simulink model "ESP_RTW"  (Simulink 8.7)
settings: Solver=ode1  SolverMode=SingleTasking  StartTime=0.0  StopTime=inf  FixedStep=0.001  RelTol=1e-3
PreLoadFcn:
  | vehicle = 'Car'; if ~length(which('cmcmd')), cmenv; end
  | ESP_RTW_bus
  | ESP_RTW_params
InitFcn:
  | vehicle = 'Car'; if ~length(which('cmcmd')), cmenv; end
  | ESP_RTW_bus
  | ESP_RTW_params
undefined symbols (not defined in the file): Area_Front, Area_Rear, ay_max_off, ay_max_on, ay_per_mu_max_off, ay_per_mu_max_on, Brake_ratio, brake_valve_ctrl_kP, cat1mode1_higher, cat1mode1_lower, cat1mode2_higher, cat1mode2_lower, cat1mode3_higher, cat1mode3_lower, cat2mode1_higher, cat2mode1_lower, cat2mode2_higher, cat2mode2_lower, cat2mode3_higher, cat2mode3_lower, delta_vel, diff_lock_fac, diff_lock_off, diff_lock_on, ESP_ctrl_kD, ESP_ctrl_kI, ESP_ctrl_kP, ESP_ctrl_restore_kI, ESP_min_throttle_fac, f_ax, f_slip, g, higherlimit_highvel, higherlimit_lowvel, highervel_fac, highervelocity_fac, InitialConditionForIntegrator, limit_acc, limit_selectlow, limit_starting, limit_vdiff, locktime_throttle, lowerlimit_highvel, lowerlimit_lowvel, lowervel_fac, lowervelocity_fac, min_throttle, MPS2KMPH, MSR_ctrl_kD, MSR_ctrl_kI, MSR_ctrl_kP, MSR_min_throttle_fac, PID_kD_sideslip, PID_kD_yawrate, PID_kI_sideslip, PID_kI_yawrate, PID_kP_sideslip, PID_kP_yawrate, RADpS2RpM, rBrake ... (+37)
libraries: CarMaker4SL x133, simulink x47, simulink_extras x6
(part 2 of 4)

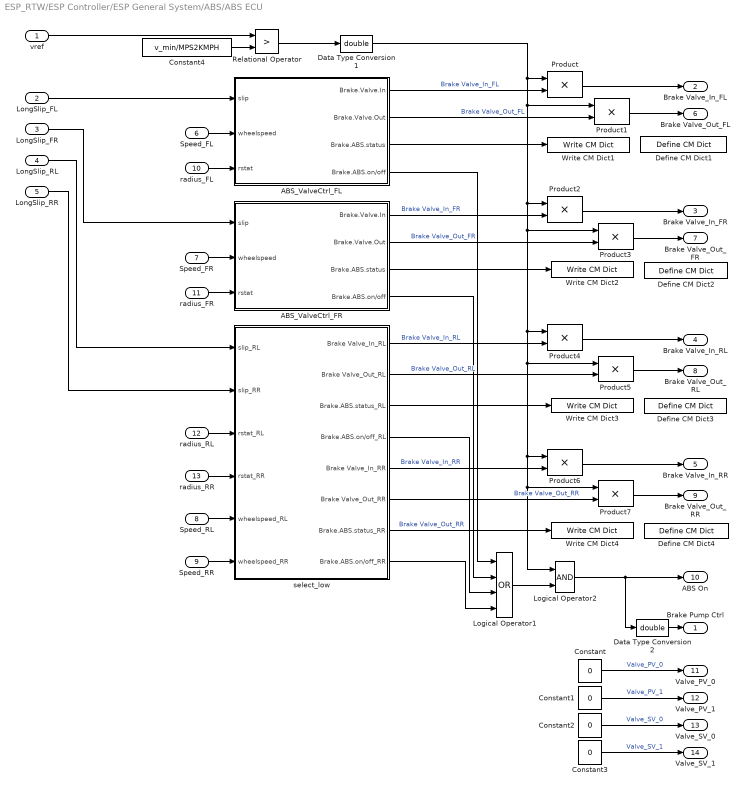
== system ESP_RTW/ESP Controller/ESP General System/ABS/ABS ECU ==
  vref : Inport
  LongSlip_FL : Inport  Port=2
  LongSlip_FR : Inport  Port=3
  LongSlip_RL : Inport  Port=4
  LongSlip_RR : Inport  Port=5
  Speed_FL : Inport  Port=6
  Speed_FR : Inport  Port=7
  Speed_RL : Inport  Port=8
  Speed_RR : Inport  Port=9
  radius_FL : Inport  Port=10
  radius_FR : Inport  Port=11
  radius_RL : Inport  Port=12
  radius_RR : Inport  Port=13
  ABS_ValveCtrl_FL : Subsystem
  ABS_ValveCtrl_FR : Subsystem
  Constant{,1..3} (4 alike) : Constant  Value=0
  Constant4 : Constant  Value=v_min/MPS2KMPH
  Data Type Conversion1 : DataTypeConversion  OutDataTypeStr=double
  Data Type Conversion2 : DataTypeConversion  OutDataTypeStr=double
  Define CM Dict1 : CarMaker4SL/Define CM Dict  xname=ESP.ABS.Status_FL  xmono=off  xtype=Char  xdvaplace=None  xnstates=4  xfirststate=0  xinitial=0
  Define CM Dict2 : CarMaker4SL/Define CM Dict  xname=ESP.ABS.Status_FR  xmono=off  xtype=Char  xdvaplace=None  xnstates=4  xfirststate=0  xinitial=0
  Define CM Dict3 : CarMaker4SL/Define CM Dict  xname=ESP.ABS.Status_RL  xmono=off  xtype=Char  xdvaplace=None  xnstates=4  xfirststate=0  xinitial=0
  Define CM Dict4 : CarMaker4SL/Define CM Dict  xname=ESP.ABS.Status_RR  xmono=off  xtype=Char  xdvaplace=None  xnstates=4  xfirststate=0  xinitial=0
  Logical Operator1 : Logic  Operator=OR  Inputs=4  AllPortsSameDT=off
  Logical Operator2 : Logic  AllPortsSameDT=off
  Product{,1..7} (8 alike) : Product  SaturateOnIntegerOverflow=on  OutDataTypeStr=Inherit: Same as first input
  Relational Operator : RelationalOperator  Operator=>
  Write CM Dict1 : CarMaker4SL/Write CM Dict  xname=ESP.ABS.Status_FL  xsync=off
  Write CM Dict2 : CarMaker4SL/Write CM Dict  xname=ESP.ABS.Status_FR  xsync=off
  Write CM Dict3 : CarMaker4SL/Write CM Dict  xname=ESP.ABS.Status_RL  xsync=off
  Write CM Dict4 : CarMaker4SL/Write CM Dict  xname=ESP.ABS.Status_RR  xsync=off
  select_low : Subsystem
  Brake Pump Ctrl : Outport
  Brake Valve_In_FL : Outport  Port=2
  Brake Valve_In_FR : Outport  Port=3
  Brake Valve_In_RL : Outport  Port=4
  Brake Valve_In_RR : Outport  Port=5
  Brake Valve_Out_FL : Outport  Port=6
  Brake Valve_Out_FR : Outport  Port=7
  Brake Valve_Out_RL : Outport  Port=8
  Brake Valve_Out_RR : Outport  Port=9
  ABS On : Outport  Port=10
  Valve_PV_0 : Outport  Port=11
  Valve_PV_1 : Outport  Port=12
  Valve_SV_0 : Outport  Port=13
  Valve_SV_1 : Outport  Port=14
  wires:
  Logical Operator2/1 -> Data Type Conversion2/1, ABS On/1
  Logical Operator1/1 -> Logical Operator2/2
  Constant3/1 -> Valve_SV_1/1  "Valve_SV_1"
  Constant2/1 -> Valve_SV_0/1  "Valve_SV_0"
  Constant1/1 -> Valve_PV_1/1  "Valve_PV_1"
  Constant/1 -> Valve_PV_0/1  "Valve_PV_0"
  vref/1 -> Relational Operator/1
  Speed_RR/1 -> select_low/6(wheelspeed_RR)
  Speed_RL/1 -> select_low/5(wheelspeed_RL)
  radius_RR/1 -> select_low/4(rstat_RR)
  radius_RL/1 -> select_low/3(rstat_RL)
  radius_FR/1 -> ABS_ValveCtrl_FR/3(rstat)
  Speed_FR/1 -> ABS_ValveCtrl_FR/2(wheelspeed)
  radius_FL/1 -> ABS_ValveCtrl_FL/3(rstat)
  Speed_FL/1 -> ABS_ValveCtrl_FL/2(wheelspeed)
  Product2/1 -> Brake Valve_In_FR/1
  Product/1 -> Brake Valve_In_FL/1
  ABS_ValveCtrl_FL/3(Brake.ABS.status) -> Write CM Dict1/1
  LongSlip_RR/1 -> select_low/2(slip_RR)
  LongSlip_RL/1 -> select_low/1(slip_RL)
  LongSlip_FR/1 -> ABS_ValveCtrl_FR/1(slip)
  LongSlip_FL/1 -> ABS_ValveCtrl_FL/1(slip)
  Product1/1 -> Brake Valve_Out_FL/1
  Product3/1 -> Brake Valve_Out_FR/1
  Product4/1 -> Brake Valve_In_RL/1
  Product5/1 -> Brake Valve_Out_RL/1
  Product6/1 -> Brake Valve_In_RR/1
  Product7/1 -> Brake Valve_Out_RR/1
  select_low/6(Brake Valve_Out_RR) -> Product7/2  "Brake Valve_Out_RR"
  select_low/5(Brake Valve_In_RR) -> Product6/2  "Brake Valve_In_RR"
  select_low/2(Brake Valve_Out_RL) -> Product5/2  "Brake Valve_Out_RL"
  select_low/1(Brake Valve_In_RL) -> Product4/2  "Brake Valve_In_RL"
  ABS_ValveCtrl_FR/2(Brake.Valve.Out) -> Product3/2  "Brake Valve_Out_FR"
  ABS_ValveCtrl_FR/1(Brake.Valve.In) -> Product2/2  "Brake Valve_In_FR"
  ABS_ValveCtrl_FL/2(Brake.Valve.Out) -> Product1/2  "Brake Valve_Out_FL"
  ABS_ValveCtrl_FL/1(Brake.Valve.In) -> Product/2  "Brake Valve_In_FL"
  Relational Operator/1 -> Data Type Conversion1/1
  Constant4/1 -> Relational Operator/2
  select_low/8(Brake.ABS.on/off_RR) -> Logical Operator1/4
  select_low/4(Brake.ABS.on/off_RL) -> Logical Operator1/3
  ABS_ValveCtrl_FR/4(Brake.ABS.on/off) -> Logical Operator1/2
  ABS_ValveCtrl_FL/4(Brake.ABS.on/off) -> Logical Operator1/1
  ABS_ValveCtrl_FR/3(Brake.ABS.status) -> Write CM Dict2/1
  select_low/3(Brake.ABS.status_RL) -> Write CM Dict3/1
  select_low/7(Brake.ABS.status_RR) -> Write CM Dict4/1  "Brake Valve_Out_RR"
  Data Type Conversion1/1 -> Product1/1, Product2/1, Product3/1, Product4/1, Product5/1, Logical Operator2/1, Product7/1, Product6/1, Product/1
  Data Type Conversion2/1 -> Brake Pump Ctrl/1

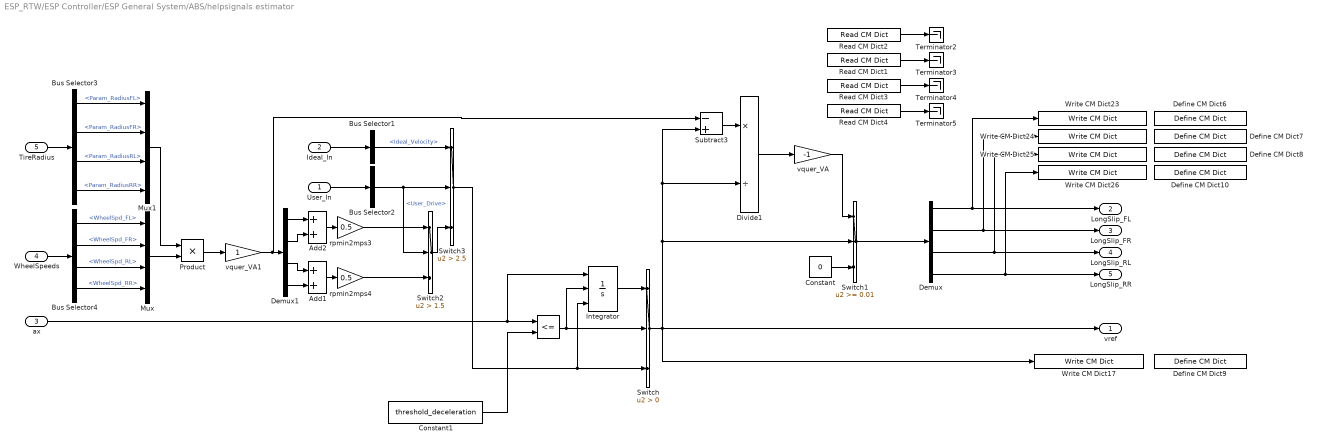
== system ESP_RTW/ESP Controller/ESP General System/ABS/helpsignals estimator ==
  User_In : Inport
  Ideal_In : Inport  Port=2
  ax : Inport  Port=3
  WheelSpeeds : Inport  Port=4
  TireRadius : Inport  Port=5
  " " : RelationalOperator  Operator=<=  OutDataTypeStr=boolean
  Add1 : Sum
  Add2 : Sum
  Bus Selector1 : BusSelector  OutputSignals=Ideal_Velocity.Ideal_Velocity
  Bus Selector2 : BusSelector  OutputSignals=User_Drive
  Bus Selector3 : BusSelector  OutputSignals=Param_RadiusFL,Param_RadiusFR,Param_RadiusRL,Param_RadiusRR
  Bus Selector4 : BusSelector  OutputSignals=WheelSpd_FL,WheelSpd_FR,WheelSpd_RL,WheelSpd_RR
  Constant : Constant  Value=0
  Constant1 : Constant  Value=threshold_deceleration
  Define CM Dict10 : CarMaker4SL/Define CM Dict  xname=ESP.ABS.LongSlip_RR  xmono=off  xtype=Double4  xdvaplace=VC  xnstates=0  xfirststate=0  xinitial=0
  Define CM Dict6 : CarMaker4SL/Define CM Dict  xname=ESP.ABS.LongSlip_FL  xmono=off  xtype=Double4  xdvaplace=VC  xnstates=0  xfirststate=0  xinitial=0
  Define CM Dict7 : CarMaker4SL/Define CM Dict  xname=ESP.ABS.LongSlip_FR  xmono=off  xtype=Double4  xdvaplace=VC  xnstates=0  xfirststate=0  xinitial=0
  Define CM Dict8 : CarMaker4SL/Define CM Dict  xname=ESP.ABS.LongSlip_RL  xmono=off  xtype=Double4  xdvaplace=VC  xnstates=0  xfirststate=0  xinitial=0
  Define CM Dict9 : CarMaker4SL/Define CM Dict  xname=ESP.ABS.v_ref  xunit=m/s  xmono=off  xtype=Double4  xdvaplace=VC  xnstates=0  xfirststate=0  xinitial=0
  Demux : Demux
  Demux1 : Demux
  Divide1 : Product  Inputs=*/
  Integrator : Integrator  ExternalReset=rising  InitialConditionSource=external
  Mux : Mux
  Mux1 : Mux
  Product : Product  RndMeth=Zero
  Read CM Dict1 : CarMaker4SL/Read CM Dict  xname=Car.LongSlipFR  xsync=off
  Read CM Dict2 : CarMaker4SL/Read CM Dict  xname=Car.LongSlipFL  xsync=off
  Read CM Dict3 : CarMaker4SL/Read CM Dict  xname=Car.LongSlipRL  xsync=off
  Read CM Dict4 : CarMaker4SL/Read CM Dict  xname=Car.LongSlipRR  xsync=off
  Subtract3 : Sum  Inputs=-+
  Switch : Switch  Criteria=u2 > Threshold
  Switch1 : Switch  Threshold=0.01
  Switch2 : Switch  Criteria=u2 > Threshold  Threshold=1.5
  Switch3 : Switch  Criteria=u2 > Threshold  Threshold=2.5
  Terminator{2..5} (4 alike) : Terminator
  Write CM Dict17 : CarMaker4SL/Write CM Dict  xname=ESP.ABS.v_ref  xsync=off
  Write CM Dict23 : CarMaker4SL/Write CM Dict  xname=ESP.ABS.LongSlip_FL  xsync=off
  Write CM Dict24 : CarMaker4SL/Write CM Dict  xname=ESP.ABS.LongSlip_FR  xsync=off
  Write CM Dict25 : CarMaker4SL/Write CM Dict  xname=ESP.ABS.LongSlip_RL  xsync=off
  Write CM Dict26 : CarMaker4SL/Write CM Dict  xname=ESP.ABS.LongSlip_RR  xsync=off
  rpmin2mps3 : Gain  Gain=0.5
  rpmin2mps4 : Gain  Gain=0.5
  vquer_VA : Gain  Gain=-1
  vquer_VA1 : Gain
  vref : Outport
  LongSlip_FL : Outport  Port=2
  LongSlip_FR : Outport  Port=3
  LongSlip_RL : Outport  Port=4
  LongSlip_RR : Outport  Port=5
  wires:
  Integrator/1 -> Switch/1
  Constant1/1 -> " "/2
  rpmin2mps4/1 -> Switch2/3
  rpmin2mps3/1 -> Switch2/1
  Bus Selector4/1 -> Mux/1  "<WheelSpd_FL>"
  Bus Selector4/2 -> Mux/2  "<WheelSpd_FR>"
  Bus Selector4/3 -> Mux/3  "<WheelSpd_RL>"
  Bus Selector4/4 -> Mux/4  "<WheelSpd_RR>"
  WheelSpeeds/1 -> Bus Selector4/1
  Bus Selector3/1 -> Mux1/1  "<Param_RadiusFL>"
  Bus Selector3/4 -> Mux1/4  "<Param_RadiusRR>"
  Bus Selector3/3 -> Mux1/3  "<Param_RadiusRL>"
  Bus Selector3/2 -> Mux1/2  "<Param_RadiusFR>"
  TireRadius/1 -> Bus Selector3/1
  Ideal_In/1 -> Bus Selector1/1
  Bus Selector1/1 -> Switch3/1  "<Ideal_Velocity>"
  Switch2/1 -> Switch3/3
  Add2/1 -> rpmin2mps3/1
  Bus Selector2/1 -> Switch3/2, Switch2/2  "<User_Drive>"
  Add1/1 -> rpmin2mps4/1
  User_In/1 -> Bus Selector2/1
  Demux1/2 -> Add2/2
  Demux1/1 -> Add2/1
  Read CM Dict4/1 -> Terminator5/1
  Read CM Dict3/1 -> Terminator4/1
  Read CM Dict1/1 -> Terminator3/1
  Read CM Dict2/1 -> Terminator2/1
  " "/1 -> Switch/2, Integrator/2
  vquer_VA1/1 -> Demux1/1, Subtract3/1
  Demux/4 -> Write CM Dict26/1, LongSlip_RR/1
  Demux/3 -> Write CM Dict25/1, LongSlip_RL/1
  Demux/2 -> Write CM Dict24/1, LongSlip_FR/1
  Demux/1 -> Write CM Dict23/1, LongSlip_FL/1
  Constant/1 -> Switch1/3
  Switch1/1 -> Demux/1
  Switch/1 -> Write CM Dict17/1, vref/1, Switch1/2, Divide1/2, Subtract3/2
  Demux1/4 -> Add1/2
  Demux1/3 -> Add1/1
  Switch3/1 -> Switch/3, Integrator/3
  ax/1 -> " "/1, Integrator/1
  vquer_VA/1 -> Switch1/1
  Divide1/1 -> vquer_VA/1
  Subtract3/1 -> Divide1/1
  Mux/1 -> Product/2
  Mux1/1 -> Product/1
  Product/1 -> vquer_VA1/1

== system ESP_RTW/ESP Controller/ESP General System/ASR/BMR ECU ==
  Throttle : Inport
  WheelVelocity [kmph] : Inport  Port=2
  User_In : Inport  Port=3
  Ideal_In : Inport  Port=4
  BMR Controller : Subsystem
  BMR logic : Subsystem
  Bus Creator : BusCreator  Inputs=8
  Bus Creator1 : BusCreator  Inputs=2
  Bus Creator2 : BusCreator  Inputs=2
  Bus Creator3 : BusCreator  Inputs=2
  Differential Lock : Subsystem
  Signal Mapping : Subsystem
  BMR On : Outport
  Brake Valves : Outport  Port=2
  Pilot Valves : Outport  Port=3
  Suctions Valves : Outport  Port=4
  Pump Ctrl : Outport  Port=5
  Diff_Torque : Outport  Port=6
  wires:
  User_In/1 -> Signal Mapping/1(User_In), Differential Lock/1(User_In), BMR Controller/1(User_In)
  BMR logic/2(BMR On) -> BMR On/1, BMR Controller/3(BMR On)
  BMR logic/1(mode) -> BMR Controller/2(mode)
  Throttle/1 -> BMR logic/5(Throttle position)
  Signal Mapping/4(v_UndrivenR) -> BMR logic/4(v_undrivenR)
  Signal Mapping/3(v_UndrivenL) -> BMR logic/3(v_undrivenL)
  Signal Mapping/2(v_DrivenR) -> BMR logic/2(v_drivenR), Differential Lock/3(v_DrivenR)
  Signal Mapping/1(v_DrivenL) -> BMR logic/1(v_drivenL), Differential Lock/2(v_DrivenL)
  Ideal_In/1 -> Signal Mapping/3(Ideal_In)
  Bus Creator3/1 -> Diff_Torque/1
  Differential Lock/2(RearDiff_Torque) -> Bus Creator3/2  "RearDiff_Torque"
  Differential Lock/1(FrontDiff_Torque) -> Bus Creator3/1  "FrontDiff_Torque"
  WheelVelocity [kmph]/1 -> Signal Mapping/2(WheelVelocity)
  Bus Creator1/1 -> Suctions Valves/1
  Bus Creator2/1 -> Pilot Valves/1
  BMR Controller/13(Pump Ctrl) -> Pump Ctrl/1  "PumpCtrl"
  BMR Controller/12(Valve_SV_1) -> Bus Creator1/2  "Valve_SV_1"
  BMR Controller/11(Valve_SV_0) -> Bus Creator1/1  "Valve_SV_0"
  BMR Controller/10(Valve_PV_1) -> Bus Creator2/2  "Valve_PV_1"
  BMR Controller/9(Valve_PV_0) -> Bus Creator2/1  "Valve_PV_0"
  BMR Controller/8(Brake Valve_Out_RR) -> Bus Creator/8  "Valve_Out_RR"
  BMR Controller/7(Brake Valve_Out_RL) -> Bus Creator/7  "Valve_Out_RL"
  BMR Controller/6(Brake Valve_Out_FR) -> Bus Creator/6  "Valve_Out_FR"
  BMR Controller/5(Brake Valve_Out_FL) -> Bus Creator/5  "Valve_Out_FL"
  BMR Controller/4(Brake Valve_In_RR) -> Bus Creator/4  "Valve_In_RR"
  BMR Controller/3(Brake Valve_In_RL) -> Bus Creator/3  "Valve_In_RL"
  BMR Controller/2(Brake Valve_In_FR) -> Bus Creator/2  "Valve_In_FR"
  BMR Controller/1(Brake Valve_In_FL) -> Bus Creator/1  "Valve_In_FL"
  Bus Creator/1 -> Brake Valves/1

== system ESP_RTW/ESP Controller/ESP General System/ASR/MSR ECU ==
  Throttle Position : Inport
  WheelVelocity [kmph] : Inport  Port=2
  User_In : Inport  Port=3
  Ideal_In : Inport  Port=4
  MSR logic : Subsystem
  MSR/Gas Controller : Subsystem
  Signal Mapping : Subsystem
  Gas_out : Outport
  MSR On : Outport  Port=2
  wires:
  MSR logic/3(hold torque) -> MSR/Gas Controller/4(hold Gas)
  MSR logic/2(reduce torque) -> MSR/Gas Controller/3(close Gas)
  MSR logic/1(Pseudo_slip) -> MSR/Gas Controller/2(Pseudo_Slip)
  Signal Mapping/4(v_UndrivenR) -> MSR logic/4(v_undrivenR)
  Signal Mapping/3(v_UndrivenL) -> MSR logic/3(v_undrivenL)
  Signal Mapping/2(v_DrivenR) -> MSR logic/2(v_drivenR)
  Signal Mapping/1(v_DrivenL) -> MSR logic/1(v_drivenL)
  Ideal_In/1 -> Signal Mapping/3(Ideal_In)
  User_In/1 -> Signal Mapping/2(User_In)
  WheelVelocity [kmph]/1 -> Signal Mapping/1(WheelVelocity)
  MSR/Gas Controller/2(Gas_Out) -> Gas_out/1
  MSR/Gas Controller/1(MSR_On) -> MSR On/1
  Throttle Position/1 -> MSR/Gas Controller/1(Throttle_position)

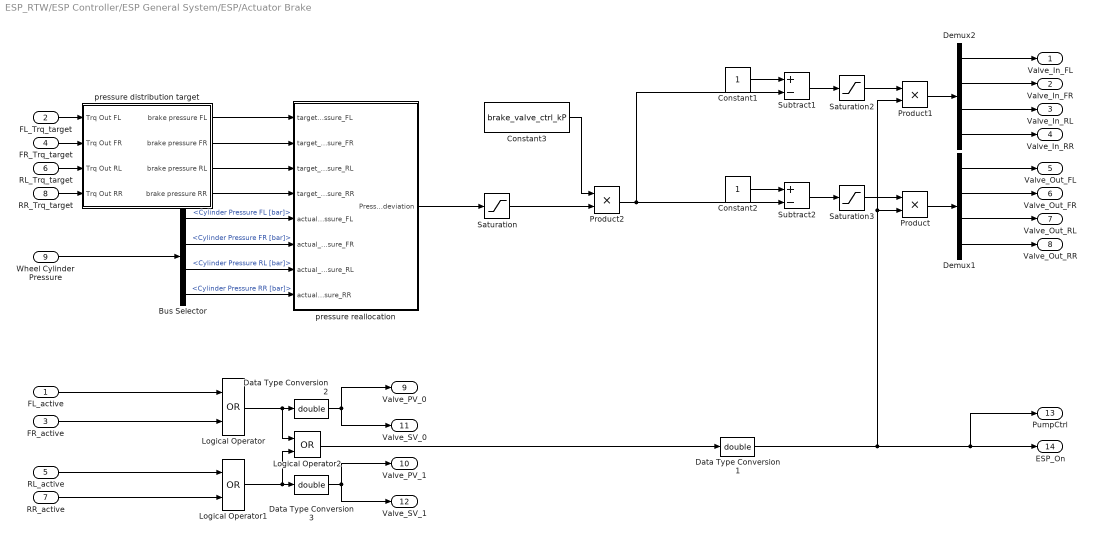
== system ESP_RTW/ESP Controller/ESP General System/ESP/Actuator Brake ==
  FL_active : Inport
  FL_Trq_target : Inport  Port=2
  FR_active : Inport  Port=3
  FR_Trq_target : Inport  Port=4
  RL_active : Inport  Port=5
  RL_Trq_target : Inport  Port=6
  RR_active : Inport  Port=7
  RR_Trq_target : Inport  Port=8
  Wheel Cylinder Pressure : Inport  Port=9
  Bus Selector : BusSelector  OutputSignals=Cylinder Pressure FL [bar],Cylinder Pressure FR [bar],Cylinder Pressure RL [bar],Cylinder Pressure RR [bar]
  Constant1 : Constant
  Constant2 : Constant
  Constant3 : Constant  Value=brake_valve_ctrl_kP
  Data Type Conversion1 : DataTypeConversion  OutDataTypeStr=double
  Data Type Conversion2 : DataTypeConversion  OutDataTypeStr=double
  Data Type Conversion3 : DataTypeConversion  OutDataTypeStr=double
  Demux1 : Demux
  Demux2 : Demux
  Logical Operator : Logic  Operator=OR  AllPortsSameDT=off
  Logical Operator1 : Logic  Operator=OR  AllPortsSameDT=off
  Logical Operator2 : Logic  Operator=OR  AllPortsSameDT=off
  Product : Product  RndMeth=Zero
  Product1 : Product  RndMeth=Zero
  Product2 : Product  RndMeth=Zero
  Saturation : Saturate  UpperLimit=500  LowerLimit=0
  Saturation2 : Saturate  UpperLimit=1  LowerLimit=0
  Saturation3 : Saturate  UpperLimit=1  LowerLimit=0
  Subtract1 : Sum  Inputs=+-
  Subtract2 : Sum  Inputs=+-
  pressure distribution target : Subsystem
  pressure reallocation : Subsystem
  Valve_In_FL : Outport
  Valve_In_FR : Outport  Port=2
  Valve_In_RL : Outport  Port=3
  Valve_In_RR : Outport  Port=4
  Valve_Out_FL : Outport  Port=5
  Valve_Out_FR : Outport  Port=6
  Valve_Out_RL : Outport  Port=7
  Valve_Out_RR : Outport  Port=8
  Valve_PV_0 : Outport  Port=9
  Valve_PV_1 : Outport  Port=10
  Valve_SV_0 : Outport  Port=11
  Valve_SV_1 : Outport  Port=12
  PumpCtrl : Outport  Port=13
  ESP_On : Outport  Port=14
  wires:
  pressure reallocation/1(Pressure deviation) -> Saturation/1
  Bus Selector/4 -> pressure reallocation/8(actual_pressure_RR)  "<Cylinder Pressure RR [bar]>"
  Bus Selector/3 -> pressure reallocation/7(actual_pressure_RL)  "<Cylinder Pressure RL [bar]>"
  Bus Selector/2 -> pressure reallocation/6(actual_pressure_FR)  "<Cylinder Pressure FR [bar]>"
  Bus Selector/1 -> pressure reallocation/5(actual_pressure_FL)  "<Cylinder Pressure FL [bar]>"
  pressure distribution target/4(brake pressure RR) -> pressure reallocation/4(target_pressure_RR)
  pressure distribution target/3(brake pressure RL) -> pressure reallocation/3(target_pressure_RL)
  pressure distribution target/2(brake pressure FR) -> pressure reallocation/2(target_pressure_FR)
  pressure distribution target/1(brake pressure FL) -> pressure reallocation/1(target_pressure_FL)
  Constant3/1 -> Product2/1
  Wheel Cylinder Pressure/1 -> Bus Selector/1
  Product1/1 -> Demux2/1
  Saturation2/1 -> Product1/1
  Product/1 -> Demux1/1
  Saturation3/1 -> Product/1
  Demux2/4 -> Valve_In_RR/1
  Demux2/3 -> Valve_In_RL/1
  Demux2/2 -> Valve_In_FR/1
  Demux2/1 -> Valve_In_FL/1
  Demux1/4 -> Valve_Out_RR/1
  Demux1/3 -> Valve_Out_RL/1
  RR_Trq_target/1 -> pressure distribution target/4(Trq Out RR)
  RL_Trq_target/1 -> pressure distribution target/3(Trq Out RL)
  Demux1/2 -> Valve_Out_FR/1
  Demux1/1 -> Valve_Out_FL/1
  Subtract2/1 -> Saturation3/1
  Subtract1/1 -> Saturation2/1
  Logical Operator2/1 -> Data Type Conversion1/1
  Logical Operator1/1 -> Logical Operator2/2, Data Type Conversion3/1
  RR_active/1 -> Logical Operator1/2
  RL_active/1 -> Logical Operator1/1
  Logical Operator/1 -> Logical Operator2/1, Data Type Conversion2/1
  FR_active/1 -> Logical Operator/2
  FL_active/1 -> Logical Operator/1
  FR_Trq_target/1 -> pressure distribution target/2(Trq Out FR)
  Constant2/1 -> Subtract2/1
  Constant1/1 -> Subtract1/1
  Saturation/1 -> Product2/2
  Product2/1 -> Subtract1/2, Subtract2/2
  FL_Trq_target/1 -> pressure distribution target/1(Trq Out FL)
  Data Type Conversion1/1 -> Product/2, Product1/2, PumpCtrl/1, ESP_On/1
  Data Type Conversion2/1 -> Valve_SV_0/1, Valve_PV_0/1
  Data Type Conversion3/1 -> Valve_SV_1/1, Valve_PV_1/1

== system ESP_RTW/ESP Controller/ESP General System/ESP/ECU ==
  ax : Inport
  Throttle Position : Inport  Port=2
  Yaw Rate : Inport  Port=3
  Steer Angle : Inport  Port=4
  Sideslip : Inport  Port=5
  mu : Inport  Port=6
  ay : Inport  Port=7
  Ideal_In : Inport  Port=8
  Vehicle Params : Inport  Port=9
  User_In : Inport  Port=10
  ECU logic : Subsystem
  Instability detectors : Subsystem
  Motor management strategy : Subsystem
  brake distribution strategy : Subsystem
  Gas_out : Outport
  FL_active : Outport  Port=2
  FL_Trq_target : Outport  Port=3
  FR_active : Outport  Port=4
  FR_Trq_target : Outport  Port=5
  RL_active : Outport  Port=6
  RL_Trq_target : Outport  Port=7
  RR_active : Outport  Port=8
  RR_Trq_target : Outport  Port=9
  wires:
  User_In/1 -> brake distribution strategy/4(User_In)
  Vehicle Params/1 -> brake distribution strategy/3(Vehicle Params), Instability detectors/7(Vehicle Params)
  Ideal_In/1 -> Instability detectors/6(Ideal_In), ECU logic/4(Ideal_In)
  mu/1 -> Instability detectors/5(mu_max), ECU logic/3(mu_max)
  Sideslip/1 -> Instability detectors/4(Sideslip)
  Instability detectors/3(motormanagement activation) -> Motor management strategy/1(activation DK)
  ay/1 -> Instability detectors/3(ay)
  Motor management strategy/1(Gas_out) -> Gas_out/1
  ax/1 -> Motor management strategy/3(ax)
  Throttle Position/1 -> Motor management strategy/2(Throttle_position)
  Instability detectors/2(YawRate corrected deviation) -> ECU logic/2(YawRate corrected deviation)
  Instability detectors/1(SideSlipAngle deviation) -> ECU logic/1(SideSlipAngle deviation)
  brake distribution strategy/8(Trq_RR_target) -> RR_Trq_target/1
  brake distribution strategy/7(RR_active) -> RR_active/1
  brake distribution strategy/6(Trq_RL_target) -> RL_Trq_target/1
  brake distribution strategy/5(RL_active) -> RL_active/1
  brake distribution strategy/4(Trq_FR_target) -> FR_Trq_target/1
  brake distribution strategy/3(FR_active) -> FR_active/1
  brake distribution strategy/2(Trq_FL_target) -> FL_Trq_target/1
  brake distribution strategy/1(FL_active) -> FL_active/1
  Yaw Rate/1 -> Instability detectors/2(Yaw Rate)
  Steer Angle/1 -> brake distribution strategy/1(Steer Angle), Instability detectors/1(Steer Angle)
  ECU logic/1(Stabilizing Torque) -> brake distribution strategy/2(Stabilizing Torque)

== system ESP_RTW/ESP Controller/ESP General System/ESP/helpsignals estimator ==
  Steer Angle : Inport
  Ideal_In : Inport  Port=2
  Vehicle Params : Inport  Port=3
  User_In : Inport  Port=4
  Bus Selector1 : BusSelector  OutputSignals=Ideal_SideSlipAngle
  Bus Selector2 : BusSelector  OutputSignals=User_estimators_on.User_SideSlip_estimator_on,User_estimators_on.User_mue_estimator_on
  Bus Selector3 : BusSelector  OutputSignals=Ideal_mu.Ideal_muFL,Ideal_mu.Ideal_muFR,Ideal_mu.Ideal_muRL,Ideal_mu.Ideal_muRR
  MinMax : MinMax  Inputs=4
  SideSlip estimator : Subsystem
  Switch : Switch  Criteria=u2 > Threshold
  Switch1 : Switch  Criteria=u2 > Threshold
  mue estimator : Subsystem
  SideslipAngle : Outport
  mu : Outport  Port=2
  wires:
  Vehicle Params/1 -> mue estimator/2(Vehicle Params)
  Bus Selector3/1 -> MinMax/1  "<Ideal_muFL>"
  Bus Selector3/4 -> MinMax/4  "<Ideal_muRR>"
  Bus Selector3/2 -> MinMax/2  "<Ideal_muFR>"
  Bus Selector3/3 -> MinMax/3  "<Ideal_muRL>"
  Ideal_In/1 -> Bus Selector1/1, SideSlip estimator/2(CarMaker_In), mue estimator/1(CarMaker_In), Bus Selector3/1
  MinMax/1 -> Switch1/3
  Switch1/1 -> mu/1
  Bus Selector2/2 -> Switch1/2  "<User_mue_estimator_on>"
  Switch/1 -> SideslipAngle/1
  SideSlip estimator/1(SideSlipAngle_estimated) -> Switch/1
  Bus Selector1/1 -> Switch/3  "<Ideal_SideSlipAngle>"
  Bus Selector2/1 -> Switch/2  "<User_SideSlip_estimator_on>"
  User_In/1 -> Bus Selector2/1
  mue estimator/1(mue_estimated) -> Switch1/1
  Steer Angle/1 -> SideSlip estimator/1(lenkwinkel)

== system ESP_RTW/ESP Controller/ESP General System/Master Controller/ABS Off ==
  ABS On : Inport
  ABS Bus : Inport  Port=2
  Bus Creator : BusCreator  Inputs=8
  Bus Creator4 : BusCreator  Inputs='Pilot Valves','Suction Valves','Brake Valves','Pump Ctrl'
  Bus Selector1 : BusSelector  OutputSignals=Valve_In_FL,Valve_In_FR,Valve_In_RL,Valve_In_RR,Valve_Out_FL,Valve_Out_FR,Valve_Out_RL,Valve_Out_RR
  Bus Selector3 : BusSelector  OutputSignals=Pilot Valves,Suction Valves,Brake Valves,Pump Ctrl
  Product{,1..7} (8 alike) : Product  RndMeth=Zero
  ABS Bus Out : Outport
  wires:
  Product7/1 -> Bus Creator/8  "Valve_Out_RR"
  Bus Selector1/8 -> Product7/2  "<Valve_Out_RR>"
  Product6/1 -> Bus Creator/7  "Valve_Out_RL"
  Bus Selector1/7 -> Product6/2  "<Valve_Out_RL>"
  Product5/1 -> Bus Creator/6  "Valve_Out_FR"
  Bus Selector1/6 -> Product5/2  "<Valve_Out_FR>"
  Product4/1 -> Bus Creator/5  "Valve_Out_FL"
  Bus Selector1/5 -> Product4/2  "<Valve_Out_FL>"
  Product3/1 -> Bus Creator/4  "Valve_In_RR"
  Bus Selector1/4 -> Product3/2  "<Valve_In_RR>"
  Product2/1 -> Bus Creator/3  "Valve_In_RL"
  Bus Selector1/3 -> Product2/2  "<Valve_In_RL>"
  Product1/1 -> Bus Creator/2  "Valve_In_FR"
  Bus Selector1/2 -> Product1/2  "<Valve_In_FR>"
  Product/1 -> Bus Creator/1  "Valve_In_FL"
  Bus Selector1/1 -> Product/2  "<Valve_In_FL>"
  ABS On/1 -> Product/1, Product1/1, Product2/1, Product3/1, Product4/1, Product5/1, Product6/1, Product7/1
  Bus Creator/1 -> Bus Creator4/3  "Brake Valves"
  Bus Selector3/4 -> Bus Creator4/4  "<Pump Ctrl>"
  Bus Selector3/3 -> Bus Selector1/1  "<Brake Valves>"
  Bus Selector3/2 -> Bus Creator4/2  "<Suction Valves>"
  Bus Selector3/1 -> Bus Creator4/1  "<Pilot Valves>"
  ABS Bus/1 -> Bus Selector3/1
  Bus Creator4/1 -> ABS Bus Out/1  "ABS Bus"

== system ESP_RTW/ESP Controller/ESP General System/Master Controller/Actuator VC ==
  VC_IN : Inport
  HSA_BrakePark : Inport  Port=2
  Gas_Out_ASR : Inport  Port=3
  Gas_Out_ESP : Inport  Port=4
  HSA_Flag : Inport  Port=5
  ASR_Flag : Inport  Port=6
  ESP_Flag : Inport  Port=7
  Bus Selector3 : BusSelector  OutputSignals=Gas,Park
  Bus Creator : BusCreator  Inputs=2
  Constant : Constant
  MinMax : MinMax  Inputs=3
  MinMax1 : MinMax  Function=max  Inputs=2
  Product : Product  RndMeth=Zero
  Subtract1 : Sum  Inputs=+-+
  Subtract2 : Sum  Inputs=+-+
  VC_OUT : Outport
  wires:
  ESP_Flag/1 -> Subtract2/2
  MinMax/1 -> Bus Creator/1  "VC_Gas"
  Bus Creator/1 -> VC_OUT/1
  MinMax1/1 -> Bus Creator/2  "VC_BrakePark"
  Product/1 -> MinMax1/2
  HSA_BrakePark/1 -> Product/2
  HSA_Flag/1 -> Product/1
  Bus Selector3/2 -> MinMax1/1  "<Park>"
  Bus Selector3/1 -> MinMax/3  "<Gas>"
  VC_IN/1 -> Bus Selector3/1
  Subtract1/1 -> MinMax/2
  Gas_Out_ASR/1 -> Subtract1/3
  ASR_Flag/1 -> Subtract1/2
  Subtract2/1 -> MinMax/1
  Gas_Out_ESP/1 -> Subtract2/3
  Constant/1 -> Subtract2/1, Subtract1/1

== system ESP_RTW/ESP Controller/ESP General System/Master Controller/User Switch ==
  ESP On : Inport
  ASR On : Inport  Port=2
  ABS On : Inport  Port=3
  HSA On : Inport  Port=4
  User In : Inport  Port=5
  Bus Creator6 : BusCreator  Inputs=3
  Bus Selector : BusSelector  OutputSignals=ASR On,MSR On,BMR On
  Bus Selector4 : BusSelector  OutputSignals=User_Switch.User_Switch_Main_off,User_Switch.User_Switch_ESP_off,User_Switch.User_Switch_ASR_off,User_Switch.User_Switch_ABS_off,User_Switch.User_Switch_HSA_off
  Constant : Constant
  Product{,1..9} (10 alike) : Product  RndMeth=Zero
  Subtract{,1..4} (5 alike) : Sum  Inputs=+-
  "ESP On " : Outport
  "ASR On " : Outport  Port=2
  "ABS On " : Outport  Port=3
  "HSA On " : Outport  Port=4
  ASRASR On : Outport  Port=5
  wires:
  Product9/1 -> "HSA On "/1  "HSA On"
  HSA On/1 -> Product9/2
  Product8/1 -> Product9/1
  Subtract4/1 -> Product8/2
  Bus Selector4/5 -> Subtract4/2  "<User_Switch_HSA_off>"
  User In/1 -> Bus Selector4/1
  Product7/1 -> "ABS On "/1  "ABS On"
  ABS On/1 -> Product7/2
  Product2/1 -> Product7/1
  Product6/1 -> Bus Creator6/3  "BMR On"
  Bus Selector/3 -> Product6/2  "<BMR On>"
  Bus Creator6/1 -> "ASR On "/1  "ASR On"
  Product5/1 -> Bus Creator6/2  "MSR On"
  Bus Selector/2 -> Product5/2  "<MSR On>"
  Product4/1 -> ASRASR On/1, Bus Creator6/1  "ASR On"
  Bus Selector/1 -> Product4/2  "<ASR On>"
  Product1/1 -> Product4/1, Product5/1, Product6/1
  Product3/1 -> "ESP On "/1  "ESP On"
  ESP On/1 -> Product3/2
  Product/1 -> Product3/1
  Subtract3/1 -> Product2/2
  Subtract2/1 -> Product1/2
  Subtract1/1 -> Product/2
  Subtract/1 -> Product2/1, Product8/1, Product1/1, Product/1
  Bus Selector4/4 -> Subtract3/2  "<User_Switch_ABS_off>"
  Bus Selector4/3 -> Subtract2/2  "<User_Switch_ASR_off>"
  Bus Selector4/2 -> Subtract1/2  "<User_Switch_ESP_off>"
  Bus Selector4/1 -> Subtract/2  "<User_Switch_Main_off>"
  Constant/1 -> Subtract/1, Subtract1/1, Subtract2/1, Subtract3/1, Subtract4/1
  ASR On/1 -> Bus Selector/1

== system ESP_RTW/ESP Controller/ESP General System/ABS/ABS ECU/ABS_ValveCtrl_FL ==
  note: EITHER ABS is switched on and  S_K is put through
      |  when S_K is becomming bigger the s_{ku}
      | OR output is 0 when S_K is smaller than {sku}_{off}
  note: Valve Control:
      | Valves are open for a predefined time window.
      | The driving time depends on a trigger criterion (LUT).
      | The treshold change for the valve driving time is
      | continously modified by a repeating sequence.
  note: Control strategy: Trigger criterion S_K
      | S_K combines wheel decceleration control with slip control
      | using weighting factors  K_z and K_\lambda
      | S_K=K_z*z_R + K_\lambda * \lambda_{rel}
      | (see p.127 in M. Burckhardt
      | Fahrwerktechnik:Radschlupfregelsysteme)
  slip : Inport
  wheelspeed : Inport  Port=2
  rstat : Inport  Port=3
  Constant : Constant
  Constant1 : Constant  Value=f_slip
  Constant3 : Constant  Value=f_ax
  Derivative : Derivative
  Duty : Subsystem
  Look-Up Table1 : Lookup  InputValues=Valve_LUTin_VA  Table=ValveIn_LUTout_VA  LookUpMeth=Interpolation-Use End Values  SaturateOnIntegerOverflow=on
  Look-Up Table2 : Lookup  InputValues=Valve_LUTin_VA  Table=ValveOut_LUTout_VA  LookUpMeth=Interpolation-Use End Values  SaturateOnIntegerOverflow=on
  Product : Product  SaturateOnIntegerOverflow=on  OutDataTypeStr=Inherit: Same as first input
  Product1 : Product  Inputs=3  SaturateOnIntegerOverflow=on  InputSameDT=on  OutDataTypeStr=Inherit: Same as first input
  Product2 : Product  SaturateOnIntegerOverflow=on  OutDataTypeStr=Inherit: Same as first input
  Rate Transition{1..4} (4 alike) : RateTransition
  Relational Operator : RelationalOperator  Operator=<  SampleTime=0.001
  Relational Operator1 : RelationalOperator  Operator=<  SampleTime=0.001
  Relay : Relay  OnSwitchValue=sku_VA  OffSwitchValue=sku_off_VA
  Sum : Sum  Inputs=|--  SaturateOnIntegerOverflow=on  InputSameDT=on  OutDataTypeStr=Inherit: Same as first input
  Sum1 : Sum  Inputs=--+  SaturateOnIntegerOverflow=on
  Zero-Order Hold : ZeroOrderHold  SampleTime=t_Sensor
  Brake.Valve.In : Outport
  Brake.Valve.Out : Outport  Port=2
  Brake.ABS.status : Outport  Port=3
  Brake.ABS.on/off : Outport  Port=4
  wires:
  Rate Transition2/1 -> Relational Operator1/1, Relational Operator/1
  Rate Transition4/1 -> Brake.ABS.on/off/1
  Rate Transition3/1 -> Relational Operator1/2
  Rate Transition1/1 -> Relational Operator/2
  Duty/1(SZ) -> Rate Transition2/1
  Constant1/1 -> Product2/1
  Derivative/1 -> Product1/1
  Product2/1 -> Sum/1
  Product1/1 -> Sum/2
  slip/1 -> Product2/2
  wheelspeed/1 -> Derivative/1
  rstat/1 -> Product1/2
  Constant3/1 -> Product1/3
  Relational Operator/1 -> Brake.Valve.In/1, Sum1/1
  Relational Operator1/1 -> Sum1/2, Brake.Valve.Out/1
  Constant/1 -> Sum1/3
  Sum1/1 -> Brake.ABS.status/1
  Sum/1 -> Zero-Order Hold/1  "S_K"
  Product/1 -> Look-Up Table2/1, Look-Up Table1/1
  Look-Up Table1/1 -> Rate Transition1/1
  Look-Up Table2/1 -> Rate Transition3/1
  Relay/1 -> Product/2, Rate Transition4/1
  Zero-Order Hold/1 -> Relay/1, Product/1

== system ESP_RTW/ESP Controller/ESP General System/ABS/ABS ECU/ABS_ValveCtrl_FR ==
  note: EITHER ABS is switched on and  S_K is put through
      |  when S_K is becomming bigger the s_{ku}
      | OR output is 0 when S_K is smaller than {sku}_{off}
  note: Valve Control:
      | Valves are open for a predefined time window.
      | The driving time depends on a trigger criterion (LUT).
      | The treshold change for the valve driving time is
      | continously modified by a repeating sequence.
  note: Control strategy: Trigger criterion S_K
      | S_K combines wheel decceleration control with slip control
      | using weighting factors  K_z and K_\lambda
      | S_K=K_z*z_R + K_\lambda * \lambda_{rel}
      | (see p.127 in M. Burckhardt
      | Fahrwerktechnik:Radschlupfregelsysteme)
  slip : Inport
  wheelspeed : Inport  Port=2
  rstat : Inport  Port=3
  Constant : Constant
  Constant1 : Constant  Value=f_slip
  Constant3 : Constant  Value=f_ax
  Derivative : Derivative
  Duty : Subsystem
  Look-Up Table1 : Lookup  InputValues=Valve_LUTin_VA  Table=ValveIn_LUTout_VA  LookUpMeth=Interpolation-Use End Values  SaturateOnIntegerOverflow=on
  Look-Up Table2 : Lookup  InputValues=Valve_LUTin_VA  Table=ValveOut_LUTout_VA  LookUpMeth=Interpolation-Use End Values  SaturateOnIntegerOverflow=on
  Product : Product  SaturateOnIntegerOverflow=on  OutDataTypeStr=Inherit: Same as first input
  Product1 : Product  Inputs=3  SaturateOnIntegerOverflow=on  InputSameDT=on  OutDataTypeStr=Inherit: Same as first input
  Product2 : Product  SaturateOnIntegerOverflow=on  OutDataTypeStr=Inherit: Same as first input
  Rate Transition{1..4} (4 alike) : RateTransition
  Relational Operator : RelationalOperator  Operator=<  SampleTime=0.001
  Relational Operator1 : RelationalOperator  Operator=<  SampleTime=0.001
  Relay : Relay  OnSwitchValue=sku_VA  OffSwitchValue=sku_off_VA
  Sum : Sum  Inputs=|--  SaturateOnIntegerOverflow=on  InputSameDT=on  OutDataTypeStr=Inherit: Same as first input
  Sum1 : Sum  Inputs=--+  SaturateOnIntegerOverflow=on
  Zero-Order Hold : ZeroOrderHold  SampleTime=t_Sensor
  Brake.Valve.In : Outport
  Brake.Valve.Out : Outport  Port=2
  Brake.ABS.status : Outport  Port=3
  Brake.ABS.on/off : Outport  Port=4
  wires:
  Rate Transition4/1 -> Brake.ABS.on/off/1
  Rate Transition3/1 -> Relational Operator1/2
  Rate Transition1/1 -> Relational Operator/2
  Rate Transition2/1 -> Relational Operator1/1, Relational Operator/1
  Constant1/1 -> Product2/1
  Derivative/1 -> Product1/1
  Product2/1 -> Sum/1
  Product1/1 -> Sum/2
  slip/1 -> Product2/2
  wheelspeed/1 -> Derivative/1
  rstat/1 -> Product1/2
  Constant3/1 -> Product1/3
  Relational Operator/1 -> Brake.Valve.In/1, Sum1/1
  Relational Operator1/1 -> Brake.Valve.Out/1, Sum1/2
  Constant/1 -> Sum1/3
  Sum1/1 -> Brake.ABS.status/1
  Sum/1 -> Zero-Order Hold/1
  Product/1 -> Look-Up Table1/1, Look-Up Table2/1
  Duty/1(SZ) -> Rate Transition2/1
  Look-Up Table1/1 -> Rate Transition1/1
  Look-Up Table2/1 -> Rate Transition3/1
  Relay/1 -> Product/2, Rate Transition4/1
  Zero-Order Hold/1 -> Relay/1, Product/1

== system ESP_RTW/ESP Controller/ESP General System/ABS/ABS ECU/select_low ==
  note: Control strategy: Trigger criterion S_K
      | S_K combines wheel decceleration control with slip control
      | using weighting factors  K_z and K_\lambda
      | S_K=K_z*z_R + K_\lambda * \lambda_{rel}
      | (see p.127 in M. Burckhardt
      | Fahrwerktechnik:Radschlupfregelsysteme)
  slip_RL : Inport
  slip_RR : Inport  Port=2
  rstat_RL : Inport  Port=3
  rstat_RR : Inport  Port=4
  wheelspeed_RL : Inport  Port=5
  wheelspeed_RR : Inport  Port=6
  ABS_ValveCtrl_rear : Subsystem
  Constant1 : Constant  Value=f_ax
  Constant2 : Constant  Value=f_slip
  Constant3 : Constant  Value=f_ax
  Constant4 : Constant  Value=f_slip
  Derivative : Derivative
  Derivative1 : Derivative
  MinMax : MinMax  Function=max  Inputs=2  SaturateOnIntegerOverflow=on  InputSameDT=on
  Product1 : Product  Inputs=3  SaturateOnIntegerOverflow=on  InputSameDT=on  OutDataTypeStr=Inherit: Same as first input
  Product2 : Product  Inputs=3  SaturateOnIntegerOverflow=on  InputSameDT=on  OutDataTypeStr=Inherit: Same as first input
  Product3 : Product  SaturateOnIntegerOverflow=on  OutDataTypeStr=Inherit: Same as first input
  Product4 : Product  SaturateOnIntegerOverflow=on  OutDataTypeStr=Inherit: Same as first input
  Sum : Sum  Inputs=|--  SaturateOnIntegerOverflow=on  InputSameDT=on  OutDataTypeStr=Inherit: Same as first input
  Sum1 : Sum  Inputs=|--  SaturateOnIntegerOverflow=on  InputSameDT=on  OutDataTypeStr=Inherit: Same as first input
  Brake Valve_In_RL : Outport
  Brake Valve_Out_RL : Outport  Port=2
  Brake.ABS.status_RL : Outport  Port=3
  Brake.ABS.on/off_RL : Outport  Port=4
  Brake Valve_In_RR : Outport  Port=5
  Brake Valve_Out_RR : Outport  Port=6
  Brake.ABS.status_RR : Outport  Port=7
  Brake.ABS.on/off_RR : Outport  Port=8
  wires:
  Constant4/1 -> Product4/1
  Constant2/1 -> Product3/1
  rstat_RR/1 -> Product1/2
  wheelspeed_RR/1 -> Derivative/1
  slip_RR/1 -> Product4/2
  ABS_ValveCtrl_rear/4(Brake.ABS.on/off) -> Brake.ABS.on/off_RL/1, Brake.ABS.on/off_RR/1
  ABS_ValveCtrl_rear/3(Brake.ABS.status) -> Brake.ABS.status_RL/1, Brake.ABS.status_RR/1
  ABS_ValveCtrl_rear/2(Brake.Valve.Out) -> Brake Valve_Out_RL/1, Brake Valve_Out_RR/1  "Brake Valve_Out_RL"
  ABS_ValveCtrl_rear/1(Brake.Valve.In) -> Brake Valve_In_RL/1, Brake Valve_In_RR/1  "Brake Valve_In_RL"
  Derivative/1 -> Product1/1
  Product4/1 -> Sum/1
  Product1/1 -> Sum/2
  Constant3/1 -> Product1/3
  Derivative1/1 -> Product2/1
  Product3/1 -> Sum1/1
  Product2/1 -> Sum1/2
  Constant1/1 -> Product2/3
  slip_RL/1 -> Product3/2
  wheelspeed_RL/1 -> Derivative1/1
  rstat_RL/1 -> Product2/2
  Sum1/1 -> MinMax/1
  Sum/1 -> MinMax/2
  MinMax/1 -> ABS_ValveCtrl_rear/1(Sk)

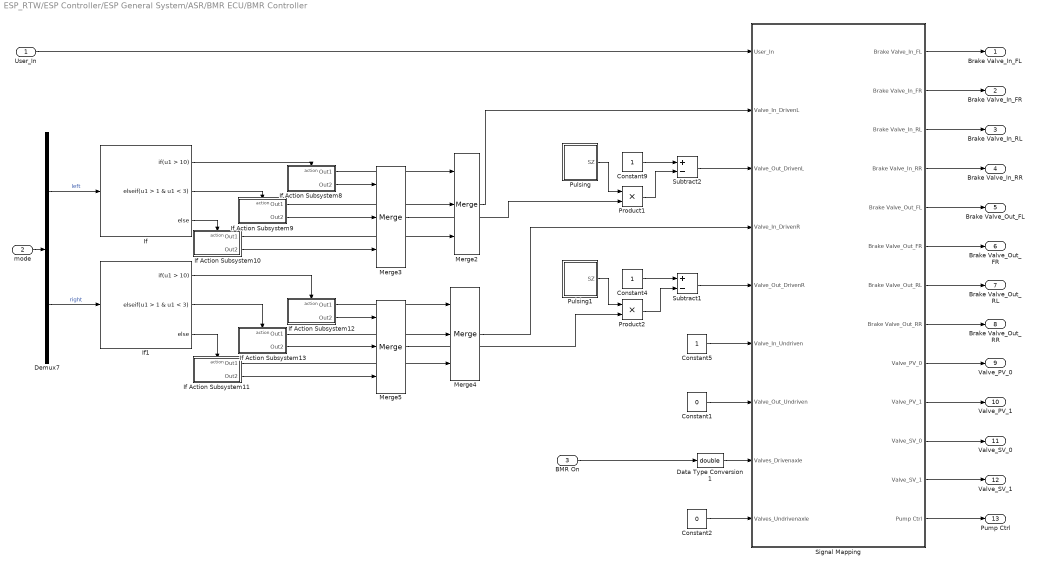
== system ESP_RTW/ESP Controller/ESP General System/ASR/BMR ECU/BMR Controller ==
  User_In : Inport
  mode : Inport  Port=2
  BMR On : Inport  Port=3
  Constant1 : Constant  Value=0
  Constant2 : Constant  Value=0
  Constant4 : Constant
  Constant5 : Constant
  Constant9 : Constant
  Data Type Conversion1 : DataTypeConversion  OutDataTypeStr=double
  Demux7 : Demux  Outputs=2
  If : If  IfExpression=u1 > 10  ElseIfExpressions=u1 > 1 & u1 < 3
  If Action Subsystem10 : Subsystem  TreatAsAtomicUnit=on
  If Action Subsystem11 : Subsystem  TreatAsAtomicUnit=on
  If Action Subsystem12 : Subsystem  TreatAsAtomicUnit=on
  If Action Subsystem13 : Subsystem  TreatAsAtomicUnit=on
  If Action Subsystem8 : Subsystem  TreatAsAtomicUnit=on
  If Action Subsystem9 : Subsystem  TreatAsAtomicUnit=on
  If1 : If  IfExpression=u1 > 10  ElseIfExpressions=u1 > 1 & u1 < 3
  Merge{2..5} (4 alike) : Merge  Inputs=3
  Product1 : Product  RndMeth=Zero
  Product2 : Product  RndMeth=Zero
  Pulsing : Subsystem
  Pulsing1 : Subsystem
  Signal Mapping : Subsystem
  Subtract1 : Sum  Inputs=+-
  Subtract2 : Sum  Inputs=+-
  Brake Valve_In_FL : Outport
  Brake Valve_In_FR : Outport  Port=2
  Brake Valve_In_RL : Outport  Port=3
  Brake Valve_In_RR : Outport  Port=4
  Brake Valve_Out_FL : Outport  Port=5
  Brake Valve_Out_FR : Outport  Port=6
  Brake Valve_Out_RL : Outport  Port=7
  Brake Valve_Out_RR : Outport  Port=8
  Valve_PV_0 : Outport  Port=9
  Valve_PV_1 : Outport  Port=10
  Valve_SV_0 : Outport  Port=11
  Valve_SV_1 : Outport  Port=12
  Pump Ctrl : Outport  Port=13
  wires:
  Pulsing/1(SZ) -> Product1/1
  Pulsing1/1(SZ) -> Product2/1
  Subtract2/1 -> Signal Mapping/3(Valve_Out_DrivenL)
  Subtract1/1 -> Signal Mapping/5(Valve_Out_DrivenR)
  User_In/1 -> Signal Mapping/1(User_In)
  Signal Mapping/13(Pump Ctrl) -> Pump Ctrl/1
  Signal Mapping/12(Valve_SV_1) -> Valve_SV_1/1
  Signal Mapping/11(Valve_SV_0) -> Valve_SV_0/1
  Signal Mapping/10(Valve_PV_1) -> Valve_PV_1/1
  Signal Mapping/9(Valve_PV_0) -> Valve_PV_0/1
  Signal Mapping/8(Brake Valve_Out_RR) -> Brake Valve_Out_RR/1
  Signal Mapping/7(Brake Valve_Out_RL) -> Brake Valve_Out_RL/1
  Signal Mapping/6(Brake Valve_Out_FR) -> Brake Valve_Out_FR/1
  Signal Mapping/5(Brake Valve_Out_FL) -> Brake Valve_Out_FL/1
  Signal Mapping/4(Brake Valve_In_RR) -> Brake Valve_In_RR/1
  Signal Mapping/3(Brake Valve_In_RL) -> Brake Valve_In_RL/1
  Signal Mapping/2(Brake Valve_In_FR) -> Brake Valve_In_FR/1
  Signal Mapping/1(Brake Valve_In_FL) -> Brake Valve_In_FL/1
  Constant2/1 -> Signal Mapping/9(Valves_Undrivenaxle)
  BMR On/1 -> Data Type Conversion1/1
  Constant1/1 -> Signal Mapping/7(Valve_Out_Undriven)
  Constant5/1 -> Signal Mapping/6(Valve_In_Undriven)
  Merge4/1 -> Signal Mapping/4(Valve_In_DrivenR)
  Merge2/1 -> Signal Mapping/2(Valve_In_DrivenL)
  mode/1 -> Demux7/1
  Product1/1 -> Subtract2/2
  Constant9/1 -> Subtract2/1
  Product2/1 -> Subtract1/2
  Constant4/1 -> Subtract1/1
  Merge5/1 -> Product2/2
  Merge3/1 -> Product1/2
  Demux7/2 -> If1/1  "right"
  If Action Subsystem11/2(Out2) -> Merge5/3
  If Action Subsystem13/2(Out2) -> Merge5/2
  If Action Subsystem12/2(Out2) -> Merge5/1
  If Action Subsystem11/1(Out1) -> Merge4/3
  If Action Subsystem13/1(Out1) -> Merge4/2
  If Action Subsystem12/1(Out1) -> Merge4/1
  If1/3 -> If Action Subsystem11/Action
  If1/2 -> If Action Subsystem13/Action
  If1/1 -> If Action Subsystem12/Action
  If Action Subsystem10/2(Out2) -> Merge3/3
  If Action Subsystem9/2(Out2) -> Merge3/2
  If Action Subsystem8/2(Out2) -> Merge3/1
  If Action Subsystem10/1(Out1) -> Merge2/3
  If Action Subsystem9/1(Out1) -> Merge2/2
  If Action Subsystem8/1(Out1) -> Merge2/1
  If/3 -> If Action Subsystem10/Action
  If/2 -> If Action Subsystem9/Action
  If/1 -> If Action Subsystem8/Action
  Demux7/1 -> If/1  "left"
  Data Type Conversion1/1 -> Signal Mapping/8(Valves_Drivenaxle)

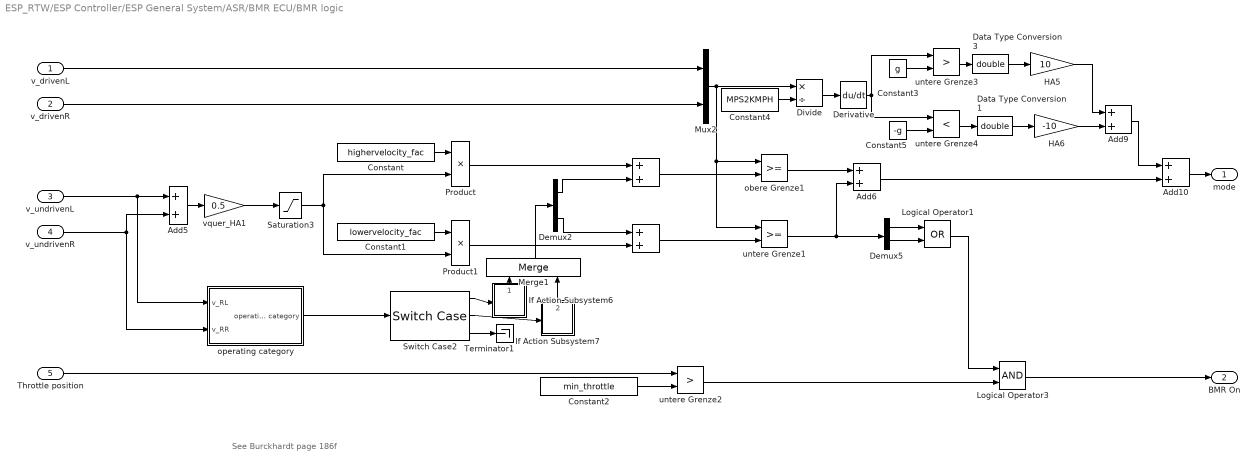
== system ESP_RTW/ESP Controller/ESP General System/ASR/BMR ECU/BMR logic ==
  note: See Burckhardt page 186f
  v_drivenL : Inport
  v_drivenR : Inport  Port=2
  v_undrivenL : Inport  Port=3
  v_undrivenR : Inport  Port=4
  Throttle position : Inport  Port=5
  " " : Sum
  "   " : Sum
  Add{5..6,9..10} (4 alike) : Sum
  Constant : Constant  Value=highervelocity_fac
  Constant1 : Constant  Value=lowervelocity_fac
  Constant2 : Constant  Value=min_throttle
  Constant3 : Constant  Value=g
  Constant4 : Constant  Value=MPS2KMPH
  Constant5 : Constant  Value=-g
  Data Type Conversion1 : DataTypeConversion  OutDataTypeStr=double
  Data Type Conversion3 : DataTypeConversion  OutDataTypeStr=double
  Demux2 : Demux  Outputs=2
  Demux5 : Demux  Outputs=2
  Derivative : Derivative
  Divide : Product  Inputs=*/
  HA5 : Gain  Gain=10
  HA6 : Gain  Gain=-10
  If Action Subsystem6 : Subsystem  TreatAsAtomicUnit=on
  If Action Subsystem7 : Subsystem  TreatAsAtomicUnit=on
  Logical Operator1 : Logic  Operator=OR  AllPortsSameDT=off
  Logical Operator3 : Logic  AllPortsSameDT=off
  Merge1 : Merge
  Mux2 : Mux  Inputs=2
  Product : Product  RndMeth=Zero
  Product1 : Product  RndMeth=Zero
  Saturation3 : Saturate  UpperLimit=inf  LowerLimit=1
  Switch Case2 : SwitchCase  CaseConditions={1,2}
  Terminator1 : Terminator
  obere Grenze1 : RelationalOperator  OutDataTypeStr=boolean
  operating category : Subsystem
  untere Grenze1 : RelationalOperator  OutDataTypeStr=boolean
  untere Grenze2 : RelationalOperator  Operator=>
  untere Grenze3 : RelationalOperator  Operator=>
  untere Grenze4 : RelationalOperator  Operator=<
  vquer_HA1 : Gain  Gain=0.5
  mode : Outport
  BMR On : Outport  Port=2
  wires:
  v_drivenL/1 -> Mux2/1
  v_drivenR/1 -> Mux2/2
  Mux2/1 -> untere Grenze1/1, obere Grenze1/1, Divide/1
  " "/1 -> untere Grenze1/2
  Constant5/1 -> untere Grenze4/2
  Constant3/1 -> untere Grenze3/2
  Constant4/1 -> Divide/2
  Constant2/1 -> untere Grenze2/2
  Constant1/1 -> Product1/1
  Constant/1 -> Product/1
  v_undrivenR/1 -> operating category/2(v_RR), Add5/2
  v_undrivenL/1 -> Add5/1, operating category/1(v_RL)
  untere Grenze2/1 -> Logical Operator3/2
  Logical Operator1/1 -> Logical Operator3/1
  Throttle position/1 -> untere Grenze2/1
  Logical Operator3/1 -> BMR On/1
  Demux5/2 -> Logical Operator1/2
  Demux5/1 -> Logical Operator1/1
  Add10/1 -> mode/1
  Add9/1 -> Add10/1
  Divide/1 -> Derivative/1
  Add6/1 -> Add10/2
  Derivative/1 -> untere Grenze3/1, untere Grenze4/1
  Data Type Conversion1/1 -> HA6/1
  Data Type Conversion3/1 -> HA5/1
  HA6/1 -> Add9/2
  HA5/1 -> Add9/1
  untere Grenze4/1 -> Data Type Conversion1/1
  untere Grenze3/1 -> Data Type Conversion3/1
  untere Grenze1/1 -> Demux5/1, Add6/2
  obere Grenze1/1 -> Add6/1
  "   "/1 -> obere Grenze1/2
  Demux2/2 -> " "/1
  Product1/1 -> " "/2
  Product/1 -> "   "/1
  Saturation3/1 -> Product/2, Product1/2
  vquer_HA1/1 -> Saturation3/1
  Add5/1 -> vquer_HA1/1
  Demux2/1 -> "   "/2
  If Action Subsystem7/1(2) -> Merge1/2
  If Action Subsystem6/1(1) -> Merge1/1
  Merge1/1 -> Demux2/1
  Switch Case2/2 -> If Action Subsystem7/Action
  Switch Case2/1 -> If Action Subsystem6/Action
  operating category/1(operating category) -> Switch Case2/1
  Switch Case2/3 -> Terminator1/1

== system ESP_RTW/ESP Controller/ESP General System/ASR/BMR ECU/Differential Lock ==
  User_In : Inport
  v_DrivenL : Inport  Port=2
  v_DrivenR : Inport  Port=3
  Abs : Abs
  Add1 : Sum  Inputs=+-
  Bus Selector1 : BusSelector  OutputSignals=User_DiffLock.User_DiffLock_Trq,User_DiffLock.User_DiffLock_on
  Bus Selector2 : BusSelector  OutputSignals=User_Drive
  Constant : Constant  Value=0
  Constant1 : Constant  Value=0
  Constant2 : Constant  Value=diff_lock_fac
  Demux : Demux  Outputs=2
  Mux : Mux  Inputs=2
  Mux1 : Mux  Inputs=2
  Mux2 : Mux  Inputs=2
  Product : Product  RndMeth=Zero
  Relay : Relay  OnSwitchValue=diff_lock_on  OffSwitchValue=diff_lock_off
  Switch1 : Switch  Criteria=u2 > Threshold
  Switch2 : Switch  Criteria=u2 > Threshold  Threshold=1.5
  Switch3 : Switch  Criteria=u2 > Threshold  Threshold=2.5
  Transfer Fcn : TransferFcn  Denominator=[0.1 1]
  FrontDiff_Torque : Outport
  RearDiff_Torque : Outport  Port=2
  wires:
  Constant2/1 -> Product/2
  Switch1/1 -> Mux/2, Mux/1, Mux1/2, Mux2/1
  Bus Selector1/1 -> Switch1/1  "<User_DiffLock_Trq>"
  Bus Selector1/2 -> Switch1/2  "<User_DiffLock_on>"
  Mux2/1 -> Switch2/3
  Constant1/1 -> Mux2/2
  Switch2/1 -> Switch3/3
  Mux1/1 -> Switch2/1
  Constant/1 -> Mux1/1
  Mux/1 -> Switch3/1
  Transfer Fcn/1 -> Switch1/3
  Switch3/1 -> Demux/1
  Demux/2 -> RearDiff_Torque/1
  Demux/1 -> FrontDiff_Torque/1
  Bus Selector2/1 -> Switch3/2, Switch2/2  "<User_Drive>"
  User_In/1 -> Bus Selector1/1, Bus Selector2/1
  v_DrivenR/1 -> Add1/2
  v_DrivenL/1 -> Add1/1
  Product/1 -> Transfer Fcn/1
  Add1/1 -> Abs/1
  Relay/1 -> Product/1
  Abs/1 -> Relay/1

== system ESP_RTW/ESP Controller/ESP General System/ASR/BMR ECU/Signal Mapping ==
  User_In : Inport
  WheelVelocity : Inport  Port=2
  Ideal_In : Inport  Port=3
  Bus Selector1 : BusSelector  OutputSignals=Ideal_Velocity.Ideal_Velocity
  Bus Selector2 : BusSelector  OutputSignals=User_Drive
  Demux1 : Demux
  Demux2 : Demux
  Mux1 : Mux
  Mux2 : Mux
  Mux3 : Mux
  Switch2 : Switch  Criteria=u2 > Threshold  Threshold=1.5
  Switch3 : Switch  Criteria=u2 > Threshold  Threshold=2.5
  v_DrivenL : Outport
  v_DrivenR : Outport  Port=2
  v_UndrivenL : Outport  Port=3
  v_UndrivenR : Outport  Port=4
  wires:
  Ideal_In/1 -> Bus Selector1/1
  Demux2/4 -> v_UndrivenR/1
  Demux2/3 -> v_UndrivenL/1
  Demux2/2 -> v_DrivenR/1
  Demux2/1 -> v_DrivenL/1
  Mux2/1 -> Switch2/1
  Mux1/1 -> Switch2/3
  Demux1/4 -> Mux2/2, Mux1/4
  Demux1/3 -> Mux2/1, Mux1/3
  Demux1/2 -> Mux3/2, Mux2/4, Mux1/2  "v_FR"
  Demux1/1 -> Mux2/3, Mux3/1, Mux1/1  "v_FL"
  Switch3/1 -> Demux2/1
  Switch2/1 -> Switch3/3
  Mux3/1 -> Switch3/1
  Bus Selector1/1 -> Mux3/4, Mux3/3  "<Ideal_Velocity>"
  Bus Selector2/1 -> Switch2/2, Switch3/2  "<User_Drive>"
  User_In/1 -> Bus Selector2/1
  WheelVelocity/1 -> Demux1/1

== system ESP_RTW/ESP Controller/ESP General System/ASR/MSR ECU/MSR logic ==
  v_drivenL : Inport
  v_drivenR : Inport  Port=2
  v_undrivenL : Inport  Port=3
  v_undrivenR : Inport  Port=4
  " " : Gain  Gain=0.5
  "   " : Gain  Gain=0.5
  Add{,1..4} (5 alike) : Sum
  Compare To Zero : simulink/Logic and Bit Operations/Compare To Zero  relop===  OutDataTypeStr=uint8
  Constant : Constant  Value=highervel_fac
  Constant1 : Constant  Value=lowervel_fac
  Demux1 : Demux  Outputs=2
  If Action Subsystem : Subsystem  TreatAsAtomicUnit=on
  If Action Subsystem1 : Subsystem  TreatAsAtomicUnit=on
  If Action Subsystem2 : Subsystem  TreatAsAtomicUnit=on
  If Action Subsystem3 : Subsystem  TreatAsAtomicUnit=on
  If Action Subsystem4 : Subsystem  TreatAsAtomicUnit=on
  If Action Subsystem5 : Subsystem  TreatAsAtomicUnit=on
  Logical Operator : Logic  AllPortsSameDT=off  OutDataTypeStr=boolean
  Merge : Merge  Inputs=6
  Product : Product  RndMeth=Zero
  Product1 : Product  RndMeth=Zero
  Saturation1 : Saturate  UpperLimit=inf  LowerLimit=1
  Saturation2 : Saturate  UpperLimit=inf  LowerLimit=1
  Subtract : Sum  Inputs=+-
  Subtract3 : Sum  Inputs=+-
  Switch Case1 : SwitchCase  CaseConditions={11,12,13,21,22,23}
  Terminator : Terminator
  lower bound : RelationalOperator  OutDataTypeStr=boolean
  operating category : Subsystem
  operating mode : Subsystem
  upper bound : RelationalOperator  OutDataTypeStr=boolean
  Pseudo_slip : Outport
  reduce torque : Outport  Port=2
  hold torque : Outport  Port=3
  wires:
  Constant1/1 -> Product1/2
  Constant/1 -> Product/1
  v_undrivenL/1 -> Add/1, operating mode/1(v_undrivenL), operating category/3(v_undrivenL)
  v_undrivenR/1 -> Add/2, operating mode/2(v_undrivenR), operating category/4(v_undrivenR)
  v_drivenR/1 -> Add1/2, operating category/2(v_drivenR)
  v_drivenL/1 -> Add1/1, operating category/1(v_drivenL)
  Product1/1 -> Add2/2
  Demux1/2 -> Add2/1
  Subtract3/1 -> Pseudo_slip/1
  Add4/1 -> upper bound/2
  Saturation2/1 -> Product/2, Subtract/2, Product1/1
  Saturation1/1 -> Subtract/1
  Subtract/1 -> Subtract3/1, lower bound/1, upper bound/1
  Logical Operator/1 -> hold torque/1  "hold moment flag"
  Compare To Zero/1 -> Logical Operator/1
  lower bound/1 -> Logical Operator/2
  upper bound/1 -> Compare To Zero/1, reduce torque/1  "reduce moment flag"
  Add2/1 -> Subtract3/2, lower bound/2
  Demux1/1 -> Add4/2
  Switch Case1/7 -> Terminator/1
  If Action Subsystem5/1(2.3) -> Merge/6
  If Action Subsystem4/1(2.2) -> Merge/5
  If Action Subsystem3/1(2.1) -> Merge/4
  If Action Subsystem2/1(1.3) -> Merge/3
  If Action Subsystem1/1(1.2) -> Merge/2
  If Action Subsystem/1(1.1) -> Merge/1
  Switch Case1/6 -> If Action Subsystem5/Action
  Switch Case1/5 -> If Action Subsystem4/Action
  Switch Case1/4 -> If Action Subsystem3/Action
  Switch Case1/3 -> If Action Subsystem2/Action
  Switch Case1/2 -> If Action Subsystem1/Action
  Merge/1 -> Demux1/1
  Switch Case1/1 -> If Action Subsystem/Action
  Add3/1 -> Switch Case1/1
  operating category/1(category) -> Add3/2
  operating mode/1(mode) -> Add3/1
  Product/1 -> Add4/1
  " "/1 -> Saturation1/1
  "   "/1 -> Saturation2/1
  Add/1 -> "   "/1
  Add1/1 -> " "/1

== system ESP_RTW/ESP Controller/ESP General System/ASR/MSR ECU/MSR/Gas Controller ==
  Throttle_position : Inport
  Pseudo_Slip : Inport  Port=2
  close Gas : Inport  Port=3
  hold Gas : Inport  Port=4
  Compare To Zero : simulink/Logic and Bit Operations/Compare To Zero  relop===  OutDataTypeStr=uint8
  Constant1 : Constant  Value=MSR_min_throttle_fac
  Constant2 : Constant  Value=min_throttle
  Data Type Conversion2 : DataTypeConversion
  Enabled Subsystem : Subsystem  TreatAsAtomicUnit=on
  Logical Operator : Logic  Operator=OR  AllPortsSameDT=off
  Logical Operator1 : Logic  AllPortsSameDT=off
  PID Controller : Subsystem
  Product2 : Product  SaturateOnIntegerOverflow=on  OutDataTypeStr=Inherit: Same as first input
  Saturation Dynamic : simulink/Discontinuities/Saturation Dynamic  OutMin=[]  OutMax=[]  OutDataTypeStr=Inherit: Same as second input  OutDataType=fixdt(1, 16)  OutScaling=2^-10  DoSatur=off
  Subtract : Sum  Inputs=-+
  Switch1 : Switch  Criteria=u2 > Threshold  Threshold=0.5
  Switch3 : Switch  Criteria=u2 > Threshold
  untere Grenze2 : RelationalOperator  Operator=>
  vquer_VA1 : Gain
  MSR_On : Outport
  Gas_Out : Outport  Port=2
  wires:
  Logical Operator1/1 -> MSR_On/1
  Logical Operator/1 -> Logical Operator1/1
  untere Grenze2/1 -> Logical Operator1/2
  Constant2/1 -> untere Grenze2/2
  Constant1/1 -> Product2/2
  Subtract/1 -> Saturation Dynamic/2
  Product2/1 -> Saturation Dynamic/3
  vquer_VA1/1 -> Saturation Dynamic/1
  Saturation Dynamic/1 -> Switch3/1
  Pseudo_Slip/1 -> PID Controller/1(u)
  PID Controller/1(y) -> Subtract/1
  Throttle_position/1 -> untere Grenze2/1, Subtract/2, vquer_VA1/1, Product2/1, Switch3/3
  Switch1/1 -> Gas_Out/1
  Enabled Subsystem/1(Out1) -> Switch1/1
  Data Type Conversion2/1 -> PID Controller/2(RESET)
  close Gas/1 -> Switch3/2, Compare To Zero/1, Logical Operator/1
  Compare To Zero/1 -> Data Type Conversion2/1
  Switch3/1 -> Enabled Subsystem/1(In1), Switch1/3
  hold Gas/1 -> Switch1/2, Logical Operator/2, Enabled Subsystem/Trigger
